simulink library "libKollege"  (R2025a)
settings: Solver=VariableStepAuto  StartTime=0.0  StopTime=10.0  RelTol=1e-3  EnableMultiTasking=on
settings Model: Creator=zatocil  LastModifiedBy=jonat
settings SolverCC: AlgebraicLoopSolver=TrustRegion
settings DataIOCC: LimitDataPoints=on  ReturnWorkspaceOutputs=off
settings OptimizationCC: LifeSpan=inf
settings DebuggingCC: UnconnectedInputMsg=warning  UnconnectedOutputMsg=warning  UnconnectedLineMsg=warning  AllowSymbolicDim=off  SFUnexpectedBacktrackingDiag=warning  SFNoUnconditionalDefaultTransitionDiag=warning  SFExecutionAtInitializationDiag=none  ArithmeticOperatorsInVariantConditions=warning
settings ModelReferenceCC: EnableRefExpFcnMdlSchedulingChecks=on  PropagateSignalLabelsOutOfModel=off
settings SFSimCC: SimUseLocalCustomCode=off  CustomCodeUndefinedFunction=UseInterfaceOnly
settings RTWCC: RTWUseLocalCustomCode=off  GPUComputeCapability=3.5
settings CodeAppCC: StateflowObjectComments=on
settings GRTTargetCC: TargetLangStandard=C89/C90 (ANSI)
settings ConfigComp: CovMetricSettings=dw  CovSaveCumulativeToWorkspaceVar=on  CovSaveSingleToWorkspaceVar=on  CovExternalEMLEnable=off

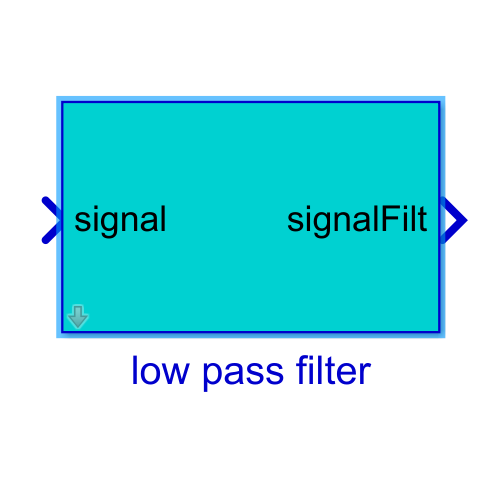
[thumbnail: Simulink's stored preview of the top-level diagram]
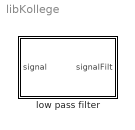
== system libKollege ==
  low pass filter : Subsystem  mask{localTFilt=1, localTsample=1}
      mask prompts: localTFilt "Filterzeitkonstante (s)"; localTsample "Abtastzeit (s)"
      mask init:
      | if localTsample <= 0
      |     error('Abtastzeit darf nicht kleiner gleich Null sein!')
      | end
      | 
      | if localTFilt <= 0
      |     error('Filterzeit darf nicht kleiner gleich Null sein!')
      | end

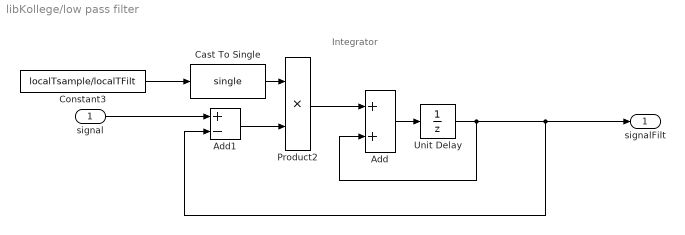
== system libKollege/low pass filter ==
  note: Integrator
  signal : Inport
  Add : Sum
  Add1 : Sum  Inputs=+-
  Cast To Single : DataTypeConversion  OutDataTypeStr=single  SaturateOnIntegerOverflow=off  RndMeth=Floor
  Constant3 : Constant  Value=localTsample/localTFilt
  Product2 : Product
  Unit Delay : UnitDelay  SampleTime=-1  HasFrameUpgradeWarning=on
  signalFilt : Outport
  wires:
  signal/1 -> Add1/1
  Unit Delay/1 -> Add/2, signalFilt/1, Add1/2
  Add1/1 -> Product2/2
  Product2/1 -> Add/1
  Add/1 -> Unit Delay/1
  Constant3/1 -> Cast To Single/1
  Cast To Single/1 -> Product2/1
